simulink model "AC_Quadcopter_Simulation_2021"  (R2021b)
settings: Solver=FixedStepAuto  StartTime=0  StopTime=50  FixedStep=0.01  MaxStep=0.06  RelTol=1e-3  EnableMultiTasking=on
InitFcn:
  | kp_roll = 2.15;
  | kd_roll = 2.5;
  | 
  | Kpmin_roll = 0.9*kp_roll;
  | Kpmax_roll = 1.05*kp_roll;
  | Kdmin_roll = 0.9*kd_roll;
  | Kdmax_roll = 1.05*kd_roll;
  | 
  | kp_pitch = 2.9;
  | kd_pitch = 3.1;
  | 
  | Kpmin_pitch = 0.9*kp_pitch;
  | Kpmax_pitch = 1.05*kp_pitch;
  | Kdmin_pitch = 0.9*kd_pitch;
  | Kdmax_pitch = 1.05*kd_pitch;
  | 
  | kp_yaw = 1;
  | kd_yaw = 2.5;
  | 
  | Kpmin_yaw = 0.8*kp_yaw;
  | Kpmax_yaw = 1.2*kp_yaw;
  | Kdmin_yaw = 0.90*kd_yaw;
  | Kdmax_yaw = 1.2*kd_yaw;
StopFcn:
  | % --- FINAL Plotting Script with Angles in Degrees ---
  | 
  | disp('Generating state tracking plots with angles in degrees...');
  | 
  | try
  |     % Assuming your timeseries variable is named 'simout'
  |     timeVector = simout.Time;
  |     dataMatrix = simout.Data;
  | 
  |     % Radian to degree conversion factor
  |     rad_to_deg = 180 / pi;
  | 
  |     % Create a new, maximized figure window for the plots
  |     figure('Name', 'Quadcopter State Tracking Performance (Degrees)', 'WindowState', 'maximized');
  | 
  |     % --- 1. Roll Tracking Plot ---
  |     subplot(2, 2, 1);
  |     hold on;
  |     % Plotting Desired (Column 5) vs. Actual (Column 1)
  |     plot(timeVector, dataMatrix(:, 5) * rad_to_deg, '--', 'LineWidth', 2);
  |     plot(timeVector, dataMatrix(:, 1) * rad_to_deg, '-', 'LineWidth', 1.5);
  |     hold off;
  |     grid on;
  |     title('Roll Angle Tracking (\phi)');
  |     xlabel('Time (s)');
  |     ylabel('Angle (deg)');
  |     legend('Desired Roll (\phi_d)', 'Actual Roll (\phi)', 'Location', 'southeast');
  | 
  |     % --- 2. Pitch Tracking Plot ---
  |     subplot(2, 2, 2);
  |     hold on;
  |     % Plotting Desired (Column 6) vs. Actual (Column 2)
  |     plot(timeVector, dataMatrix(:, 6) * rad_to_deg, '--', 'LineWidth', 2);
  |     plot(timeVector, dataMatrix(:, 2) * rad_to_deg, '-', 'LineWidth', 1.5);
  |     hold off;
  |     grid on;
  |     title('Pitch Angle Tracking (\theta)');
  |     xlabel('Time (s)');
  |     ylabel('Angle (deg)');
  |     legend('Desired Pitch (\theta_d)', 'Actual Pitch (\theta)', 'Location', 'southeast');
  | 
  |     % --- 3. Yaw Tracking Plot ---
  |     subplot(2, 2, 3);
  |     hold on;
  |     % Plotting Desired (Column 7) vs. Actual (Column 3)
  |     plot(timeVector, dataMatrix(:, 7) * rad_to_deg, '--', 'LineWidth', 2);
  |     plot(timeVector, dataMatrix(:, 3) * rad_to_deg, '-', 'LineWidth', 1.5);
  |     hold off;
  |     grid on;
  |     title('Yaw Angle Tracking (\psi)');
  |     xlabel('Time (s)');
  |     ylabel('Angle (deg)');
  |     legend('Desired Yaw (\psi_d)', 'Actual Yaw (\psi)', 'Location', 'southeast');
  | 
  |     % --- 4. Altitude Tracking Plot ---
  |     subplot(2, 2, 4);
  |     hold on;
  |     % Plotting Desired (Column 8) vs. Actual (Column 4)
  |     plot(timeVector, dataMatrix(:, 8), '--', 'LineWidth', 2);
  |     plot(timeVector, dataMatrix(:, 4), '-', 'LineWidth', 1.5);
  |     hold off;
  |     grid on;
  |     title('Altitude Tracking (Z)');
  |     xlabel('Time (s)');
  |     ylabel('Position (m)');
  |     legend('Desired Altitude (Z_d)', 'Actual Altitude (Z)', 'Location', 'southeast');
  | 
  |     sgtitle('Quadcopter State Tracking Performance', 'FontSize', 16, 'FontWeight', 'bold');
  |     disp('Plots generated successfully with units in degrees.');
  | 
  | catch ME
  |     warning('Error during plotting: %s', ME.message);
  |     warning('Please ensure the variable ''simout'' exists in the workspace.');
  | end
model workspace (MAT data in the model file):
  Sig = Simulink.Signal
  Sig.DataType = 'auto'
  Sig.Dimensions = -1
  Sig.DimensionsMode = 'auto'
  Sig.Complexity = 'auto'
  Sig.SampleTime = -1
  Sig.SamplingMode = 'auto'
undefined symbols (not defined in the file): IC, quadModel
libraries: simulink x4, fuzblock x3, slpidlib x3
Description:
  | This is a configurable quadcopter simulation.
  | This Simulink model demonstates attitude control.
  | 
  | Additional quadcopter modeling and simulation materials available at:
  | github.com/dch33/Quad-Sim
  | 
  | Copyright (C) 2014 D. Hartman, K. Landis, S. Moreno, J. Kim, M. Mehrer
  | 
  | License:
  |     This program is free software: you can redistribute it and/or modify
  |     it under the terms of the GNU LESSER GENERAL PUBLIC LICENSE as published by
  |     the Free Software Foundation, either version 3 of the License, or
  |     (at your option) any later version.
  | 
  |     This program is distributed in the hope that it will be useful,
  |     but WITHOUT ANY WARRANTY; without even the implied warranty of
  |     MERCHANTABILITY or FITNESS FOR A PARTICULAR PURPOSE.  See the
  |     GNU General Public License for more details.
  | 
  |     You should have received a copy of the GNU LESSER GENERAL PUBLIC LICENSE
  |     along with this program.  If not, see <http://www.gnu.org/licenses/>.
settings Model: ModifiedComment=hp -- Sun Aug 31 10:33:41 2025 -- Version 21.0  Creator=David Hartman  LastModifiedBy=hp
settings Model: ModifiedHistory=|
  | hp -- Sun Aug 31 10:33:41 2025 -- Version 21.0
  | 
  | davidhartman -- Fri Jun 06 23:19:51 2014 -- Version 1.5
  | 
  | 
  | davidhartman -- Fri Jun 06 22:53:10 2014 -- Version 1.3
settings SolverCC: AlgebraicLoopSolver=TrustRegion  AutoInsertRateTranBlk=on
settings DataIOCC: SaveFormat=Array  SignalLogging=off  ReturnWorkspaceOutputs=off
settings OptimizationCC: DefaultParameterBehavior=Inlined  LifeSpan=inf
settings DebuggingCC: UnderspecifiedInitializationDetection=Classic  MergeDetectMultiDrivingBlocksExec=none  SolverPrmCheckMsg=warning  UniqueDataStoreMsg=warning  StateNameClashWarn=warning  StrictBusMsg=WarnOnBusTreatedAsVector  SFUnexpectedBacktrackingDiag=warning  SFNoUnconditionalDefaultTransitionDiag=warning  SFExecutionAtInitializationDiag=none  ArithmeticOperatorsInVariantConditions=warning
settings HardwareCC: ProdBitPerPointer=32  ProdBitPerSizeT=32  ProdBitPerPtrDiffT=32  ProdLargestAtomicFloat=None  ProdIntDivRoundTo=Undefined  ProdEndianess=Unspecified  ProdWordSize=32  ProdHWDeviceType=32-bit Generic
settings ModelReferenceCC: EnableRefExpFcnMdlSchedulingChecks=off  PropagateSignalLabelsOutOfModel=off
settings SFSimCC: SimUseLocalCustomCode=off  CustomCodeUndefinedFunction=UseInterfaceOnly
settings RTWCC: RTWUseLocalCustomCode=off  DLArmComputeVersion=20.02.1
settings CodeAppCC: StateflowObjectComments=on
settings GRTTargetCC: TargetLangStandard=C89/C90 (ANSI)
settings ConfigComp: CovMetricSettings=dw  CovSaveCumulativeToWorkspaceVar=on  CovSaveSingleToWorkspaceVar=on  CovExternalEMLEnable=off

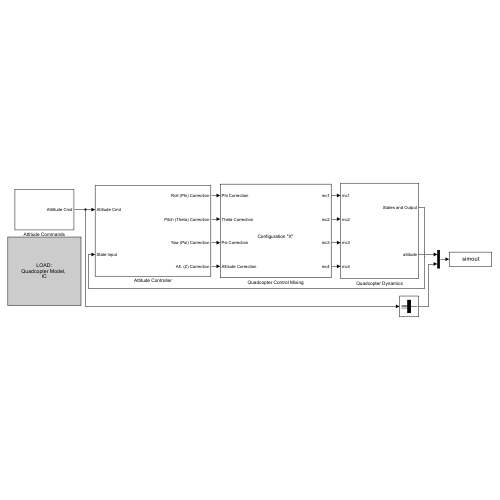
[thumbnail: Simulink's stored preview of the top-level diagram]
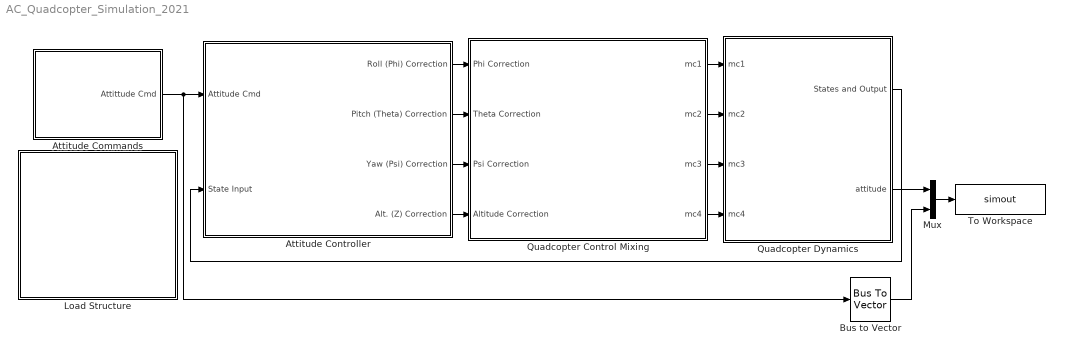
== system AC_Quadcopter_Simulation_2021 ==
  Attitude Commands : Subsystem
  Attitude Controller : Subsystem
  Bus to Vector : BusToVector
  Load Structure : Subsystem
      settings: OpenFcn=|
      | uiopen('load')
      | if ((exist('IC')==1) && (exist('quadModel')==1) && (exist('path')==1))
      | set_param(bdroot, 'SimulationCommand', 'update')
      | end
      mask Display: fprintf('LOAD:\nQuadcopter Model, \nIC')
  Mux : Mux  Inputs=2
  Quadcopter Control Mixing : Subsystem
      mask Display:
      | modelLoaded = evalin('base','exist(''quadModel'',''var'')');
      | if (modelLoaded==1)
      |     if (evalin('base','quadModel.plusConfig'))
      |     fprintf([' \n' ' \n'  'Configuration "+"']);
      |     else if (~evalin('base','quadModel.plusConfig'))
      |         fprintf([' \n' ' \n' 'Configuration "X"']);
      |         end
      |     end
      | else
      |     fprintf([' \n' ' \n'  'Model Not Loaded']);
      | end
  Quadcopter Dynamics : Subsystem
  To Workspace : ToWorkspace  VariableName=simout  SaveFormat=Timeseries  SampleTime=-1
  wires:
  Quadcopter Control Mixing/1(mc1) -> Quadcopter Dynamics/1(mc1)
  Quadcopter Dynamics/1(States and Output) -> Attitude Controller/2(State Input)
  Quadcopter Control Mixing/4(mc4) -> Quadcopter Dynamics/4(mc4)
  Quadcopter Control Mixing/2(mc2) -> Quadcopter Dynamics/2(mc2)
  Quadcopter Control Mixing/3(mc3) -> Quadcopter Dynamics/3(mc3)
  Attitude Commands/1(Attittude Cmd) -> Bus to Vector/1, Attitude Controller/1(Attitude Cmd)
  Attitude Controller/1(Roll (Phi) Correction) -> Quadcopter Control Mixing/1(Phi Correction)
  Attitude Controller/2(Pitch (Theta) Correction) -> Quadcopter Control Mixing/2(Theta Correction)
  Attitude Controller/3(Yaw (Psi) Correction) -> Quadcopter Control Mixing/3(Psi Correction)
  Attitude Controller/4(Alt. (Z) Correction) -> Quadcopter Control Mixing/4(Altitude Correction)
  Quadcopter Dynamics/2(attitude) -> Mux/1
  Mux/1 -> To Workspace/1
  Bus to Vector/1 -> Mux/2

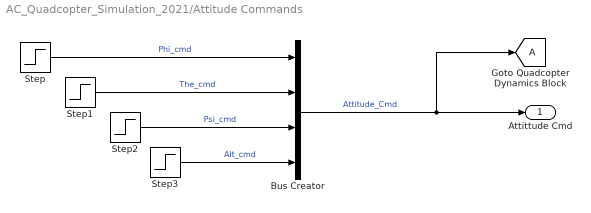
== system AC_Quadcopter_Simulation_2021/Attitude Commands ==
  Bus Creator : BusCreator  Inputs=4
  Step : Step  Time=4  After=-10*pi/180  SampleTime=0
  Step1 : Step  After=10*pi/180  SampleTime=0
  Step2 : Step  Time=7  After=45*pi/180  SampleTime=0
  Step3 : Step  Time=0  Before=10*0.3048  After=10*0.3048  SampleTime=0
  Attittude Cmd : Outport
  tag scope: A=global
  wires:
  Bus Creator/1 -> Attittude Cmd/1, [A]  "Attitude_Cmd"
  Step3/1 -> Bus Creator/4  "Alt_cmd"
  Step2/1 -> Bus Creator/3  "Psi_cmd"
  Step1/1 -> Bus Creator/2  "The_cmd"
  Step/1 -> Bus Creator/1  "Phi_cmd"

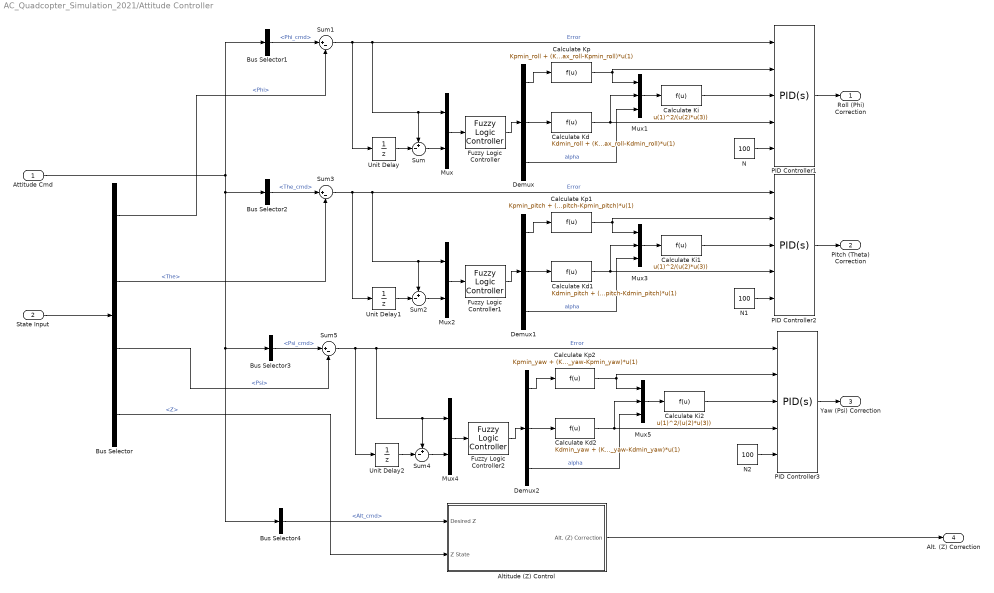
== system AC_Quadcopter_Simulation_2021/Attitude Controller ==
  Attitude Cmd : Inport
  State Input : Inport  Port=2
  Altitude (Z) Control : Subsystem  mask{Kpz=2, Kiz=1.1, Kdz=3.3, LimitOutput=on, USat=1, LSat=-1, GOffset=(sqrt((quadModel.mass*quadModel.g)/(4*quadModel.ct))-quadModel.b)/quadModel.cr}
      mask prompts: Kpz "Kp"; Kiz "Ki"; Kdz "Kd"; LimitOutput "Integral Saturation?"; USat "Upper saturation limit:"; LSat "Lower saturation limit:"; GOffset "Gravity Feedforward"
      mask help:
      | Adjust PID controller gains through this mask interface, or "look under mask" for more detailed adjustments.
      |
      | Note: Gravity Offset will not appear on block face as a value until simulation is run if it is the result of a formula involving the quadcopter model parameters.
      mask TypeOptions Kpz: Kpz/Gain
      mask TypeOptions Kiz: Kiz/Gain
      mask TypeOptions Kdz: Kdz/Gain
      mask TypeOptions LimitOutput:
      | Integrator
      | Limited/LimitOutput
      mask TypeOptions USat:
      | Integrator
      | Limited/UpperSaturationLimit
      mask TypeOptions LSat:
      | Integrator
      | Limited/LowerSaturationLimit
      mask TypeOptions GOffset: Gravity Offset (Level Flight)/Value
      mask Display:
      | fprintf(['Kp = ' num2str(Kpz) '\n' ...
      |     'Ki = ' num2str(Kiz) '\n' ...
      |     'Kd = ' num2str(Kdz) '\n' ...
      |     'Integral Saturation: ' LimitOutput]);
      | if strcmp(LimitOutput,'on')
      |     fprintf([' \n' ' \n' ' \n' ' \n' ' \n' '\n' ...
      |         'Limits: ' num2str(USat) ' to ' num2str(LSat)]);
      | end
  Bus Selector : BusSelector  OutputSignals=Phi,The,Psi,Z
  Bus Selector1 : BusSelector  OutputSignals=Phi_cmd
  Bus Selector2 : BusSelector  OutputSignals=The_cmd
  Bus Selector3 : BusSelector  OutputSignals=Psi_cmd
  Bus Selector4 : BusSelector  OutputSignals=Alt_cmd
  Calculate Kd : Fcn  Expr=Kdmin_roll + (Kdmax_roll-Kdmin_roll)*u(1)
  Calculate Kd1 : Fcn  Expr=Kdmin_pitch + (Kdmax_pitch-Kdmin_pitch)*u(1)
  Calculate Kd2 : Fcn  Expr=Kdmin_yaw + (Kdmax_yaw-Kdmin_yaw)*u(1)
  Calculate Ki : Fcn  Expr=u(1)^2/(u(2)*u(3))
  Calculate Ki1 : Fcn  Expr=u(1)^2/(u(2)*u(3))
  Calculate Ki2 : Fcn  Expr=u(1)^2/(u(2)*u(3))
  Calculate Kp : Fcn  Expr=Kpmin_roll + (Kpmax_roll-Kpmin_roll)*u(1)
  Calculate Kp1 : Fcn  Expr=Kpmin_pitch + (Kpmax_pitch-Kpmin_pitch)*u(1)
  Calculate Kp2 : Fcn  Expr=Kpmin_yaw + (Kpmax_yaw-Kpmin_yaw)*u(1)
  Demux : Demux  Outputs=3
  Demux1 : Demux  Outputs=3
  Demux2 : Demux  Outputs=3
  Fuzzy Logic Controller : fuzblock/Fuzzy Logic  Controller  FIS='PID_Fuzzy.fis'  OutputSampleNumber=101  DataType=double  FuzzifiedInputs=off  RuleFiringStrengths=off  RuleOutputs=off  AggregatedOutputs=off  SimulateUsing=Interpreted execution  OutOfRangeInputValueMessage=warning  NoRuleFiredMessage=warning  EmptyOutputFuzzySetMessage=warning
  Fuzzy Logic Controller1 : fuzblock/Fuzzy Logic  Controller  FIS='PID_Fuzzy.fis'  OutputSampleNumber=101  DataType=double  FuzzifiedInputs=off  RuleFiringStrengths=off  RuleOutputs=off  AggregatedOutputs=off  SimulateUsing=Interpreted execution  OutOfRangeInputValueMessage=warning  NoRuleFiredMessage=warning  EmptyOutputFuzzySetMessage=warning
  Fuzzy Logic Controller2 : fuzblock/Fuzzy Logic  Controller  FIS='PID_Fuzzy.fis'  OutputSampleNumber=101  DataType=double  FuzzifiedInputs=off  RuleFiringStrengths=off  RuleOutputs=off  AggregatedOutputs=off  SimulateUsing=Interpreted execution  OutOfRangeInputValueMessage=warning  NoRuleFiredMessage=warning  EmptyOutputFuzzySetMessage=warning
  Mux : Mux  Inputs=2
  Mux1 : Mux  Inputs=3
  Mux2 : Mux  Inputs=2
  Mux3 : Mux  Inputs=3
  Mux4 : Mux  Inputs=2
  Mux5 : Mux  Inputs=3
  N : Constant  Value=100
  N1 : Constant  Value=100
  N2 : Constant  Value=100
  PID Controller1 : slpidlib/PID Controller  Controller=PID  Form=Parallel  TimeDomain=Continuous-time  UseExternalTs=off  SampleTime=-1  IntegratorMethod=Forward Euler  FilterMethod=Forward Euler  ControllerParametersSource=external  P=0.6*4.6737  I=1.2*4.6737/3.26  D=0.6*4.6737*3.26/8  N=100  UseFilter=on  TunerSelectOption=Transfer Function Based (PID Tuner App)  InitialConditionSource=internal  InitialConditionForIntegrator=0  InitialConditionForFilter=0  DifferentiatorICPrevScaledInput=0  ExternalReset=none  TrackingMode=off  Kt=1  LimitOutput=off  SatLimitsSource=internal  UpperSaturationLimit=inf  LowerSaturationLimit=-inf  LinearizeAsGain=on  AntiWindupMode=none  Kb=1  POutMin=[]  POutMax=[]  IOutMin=[]  IOutMax=[]  DOutMin=[]  DOutMax=[]  NOutMin=[]  NOutMax=[]  SumOutMin=[]  SumOutMax=[]  SaturationOutMin=[]  SaturationOutMax=[]  PParamMin=[]  PParamMax=[]  IParamMin=[]  IParamMax=[]  DParamMin=[]  DParamMax=[]  NParamMin=[]  NParamMax=[]  KbParamMin=[]  KbParamMax=[]  KtParamMin=[]  KtParamMax=[]  KbOutMin=[]  KbOutMax=[]  KtOutMin=[]  KtOutMax=[]  IntegratorOutMin=[]  IntegratorOutMax=[]  FilterOutMin=[]  FilterOutMax=[]  SumI1OutMin=[]  SumI1OutMax=[]  SumI2OutMin=[]  SumI2OutMax=[]  SumI3OutMin=[]  SumI3OutMax=[]  SumI4OutMin=[]  SumI4OutMax=[]  SumDOutMin=[]  SumDOutMax=[]  DifferentiatorOutMin=[]  DifferentiatorOutMax=[]  FilterDiffOutCoefMin=[]  FilterDiffOutCoefMax=[]  ReciprocalOutMin=[]  ReciprocalOutMax=[]  SumDenOutMin=[]  SumDenOutMax=[]  SumNumOutMin=[]  SumNumOutMax=[]  DivideOutMin=[]  DivideOutMax=[]  UdiffTsProdOutMin=[]  UdiffTsProdOutMax=[]  NTsProdOutMin=[]  NTsProdOutMax=[]  UintegralTsProdOutMin=[]  UintegralTsProdOutMax=[]  UngainTsProdOutMin=[]  UngainTsProdOutMax=[]  IntegratorContinuousStateAttributes=''  IntegratorStateMustResolveToSignalObject=off  IntegratorRTWStateStorageClass=Auto  FilterContinuousStateAttributes=''  FilterStateMustResolveToSignalObject=off  FilterRTWStateStorageClass=Auto  ParallelPVariant=ExternalParameters  IdealPVariant=Disabled  IVariant=ExternalParameters  DVariant=ExternalParameters  IntegratorVariant=Continuous  SatVariant=Disabled  AWVariant=Passthrough  PCopyVariant=Disabled  TRVariant=Disabled  FdbkBlocksVariant=Forward  IdealPFdbkVariant=Disabled  SatFdbkVariant=Disabled  DerivativeFilterVariant=ContFilter  NVariant=ExternalParameters  NCopyVariant=Disabled  FilterICVariant=InternalICsFilter  IntegratorICVariant=InternalICs  ExternalResetVariant=Disabled  TRSumVariant=Passthrough  SumFdbkVariant=Disabled  SumVariant=Sum_PID  TsampFilterVariant=InternalTs  TsampNgainVariant=Passthrough  TsampIntegralVariant=Disabled_SignalSpec  ExternalSaturationOutDataTypeStr=Inherit: Same as second input
  PID Controller2 : slpidlib/PID Controller  Controller=PID  Form=Parallel  TimeDomain=Continuous-time  UseExternalTs=off  SampleTime=-1  IntegratorMethod=Forward Euler  FilterMethod=Forward Euler  ControllerParametersSource=external  P=0.6*4.6737  I=1.2*4.6737/3.26  D=0.6*4.6737*3.26/8  N=100  UseFilter=on  TunerSelectOption=Transfer Function Based (PID Tuner App)  InitialConditionSource=internal  InitialConditionForIntegrator=0  InitialConditionForFilter=0  DifferentiatorICPrevScaledInput=0  ExternalReset=none  TrackingMode=off  Kt=1  LimitOutput=off  SatLimitsSource=internal  UpperSaturationLimit=inf  LowerSaturationLimit=-inf  LinearizeAsGain=on  AntiWindupMode=none  Kb=1  POutMin=[]  POutMax=[]  IOutMin=[]  IOutMax=[]  DOutMin=[]  DOutMax=[]  NOutMin=[]  NOutMax=[]  SumOutMin=[]  SumOutMax=[]  SaturationOutMin=[]  SaturationOutMax=[]  PParamMin=[]  PParamMax=[]  IParamMin=[]  IParamMax=[]  DParamMin=[]  DParamMax=[]  NParamMin=[]  NParamMax=[]  KbParamMin=[]  KbParamMax=[]  KtParamMin=[]  KtParamMax=[]  KbOutMin=[]  KbOutMax=[]  KtOutMin=[]  KtOutMax=[]  IntegratorOutMin=[]  IntegratorOutMax=[]  FilterOutMin=[]  FilterOutMax=[]  SumI1OutMin=[]  SumI1OutMax=[]  SumI2OutMin=[]  SumI2OutMax=[]  SumI3OutMin=[]  SumI3OutMax=[]  SumI4OutMin=[]  SumI4OutMax=[]  SumDOutMin=[]  SumDOutMax=[]  DifferentiatorOutMin=[]  DifferentiatorOutMax=[]  FilterDiffOutCoefMin=[]  FilterDiffOutCoefMax=[]  ReciprocalOutMin=[]  ReciprocalOutMax=[]  SumDenOutMin=[]  SumDenOutMax=[]  SumNumOutMin=[]  SumNumOutMax=[]  DivideOutMin=[]  DivideOutMax=[]  UdiffTsProdOutMin=[]  UdiffTsProdOutMax=[]  NTsProdOutMin=[]  NTsProdOutMax=[]  UintegralTsProdOutMin=[]  UintegralTsProdOutMax=[]  UngainTsProdOutMin=[]  UngainTsProdOutMax=[]  IntegratorContinuousStateAttributes=''  IntegratorStateMustResolveToSignalObject=off  IntegratorRTWStateStorageClass=Auto  FilterContinuousStateAttributes=''  FilterStateMustResolveToSignalObject=off  FilterRTWStateStorageClass=Auto  ParallelPVariant=ExternalParameters  IdealPVariant=Disabled  IVariant=ExternalParameters  DVariant=ExternalParameters  IntegratorVariant=Continuous  SatVariant=Disabled  AWVariant=Passthrough  PCopyVariant=Disabled  TRVariant=Disabled  FdbkBlocksVariant=Forward  IdealPFdbkVariant=Disabled  SatFdbkVariant=Disabled  DerivativeFilterVariant=ContFilter  NVariant=ExternalParameters  NCopyVariant=Disabled  FilterICVariant=InternalICsFilter  IntegratorICVariant=InternalICs  ExternalResetVariant=Disabled  TRSumVariant=Passthrough  SumFdbkVariant=Disabled  SumVariant=Sum_PID  TsampFilterVariant=InternalTs  TsampNgainVariant=Passthrough  TsampIntegralVariant=Disabled_SignalSpec  ExternalSaturationOutDataTypeStr=Inherit: Same as second input
  PID Controller3 : slpidlib/PID Controller  Controller=PID  Form=Parallel  TimeDomain=Continuous-time  UseExternalTs=off  SampleTime=-1  IntegratorMethod=Forward Euler  FilterMethod=Forward Euler  ControllerParametersSource=external  P=0.6*4.6737  I=1.2*4.6737/3.26  D=0.6*4.6737*3.26/8  N=100  UseFilter=on  TunerSelectOption=Transfer Function Based (PID Tuner App)  InitialConditionSource=internal  InitialConditionForIntegrator=0  InitialConditionForFilter=0  DifferentiatorICPrevScaledInput=0  ExternalReset=none  TrackingMode=off  Kt=1  LimitOutput=off  SatLimitsSource=internal  UpperSaturationLimit=inf  LowerSaturationLimit=-inf  LinearizeAsGain=on  AntiWindupMode=none  Kb=1  POutMin=[]  POutMax=[]  IOutMin=[]  IOutMax=[]  DOutMin=[]  DOutMax=[]  NOutMin=[]  NOutMax=[]  SumOutMin=[]  SumOutMax=[]  SaturationOutMin=[]  SaturationOutMax=[]  PParamMin=[]  PParamMax=[]  IParamMin=[]  IParamMax=[]  DParamMin=[]  DParamMax=[]  NParamMin=[]  NParamMax=[]  KbParamMin=[]  KbParamMax=[]  KtParamMin=[]  KtParamMax=[]  KbOutMin=[]  KbOutMax=[]  KtOutMin=[]  KtOutMax=[]  IntegratorOutMin=[]  IntegratorOutMax=[]  FilterOutMin=[]  FilterOutMax=[]  SumI1OutMin=[]  SumI1OutMax=[]  SumI2OutMin=[]  SumI2OutMax=[]  SumI3OutMin=[]  SumI3OutMax=[]  SumI4OutMin=[]  SumI4OutMax=[]  SumDOutMin=[]  SumDOutMax=[]  DifferentiatorOutMin=[]  DifferentiatorOutMax=[]  FilterDiffOutCoefMin=[]  FilterDiffOutCoefMax=[]  ReciprocalOutMin=[]  ReciprocalOutMax=[]  SumDenOutMin=[]  SumDenOutMax=[]  SumNumOutMin=[]  SumNumOutMax=[]  DivideOutMin=[]  DivideOutMax=[]  UdiffTsProdOutMin=[]  UdiffTsProdOutMax=[]  NTsProdOutMin=[]  NTsProdOutMax=[]  UintegralTsProdOutMin=[]  UintegralTsProdOutMax=[]  UngainTsProdOutMin=[]  UngainTsProdOutMax=[]  IntegratorContinuousStateAttributes=''  IntegratorStateMustResolveToSignalObject=off  IntegratorRTWStateStorageClass=Auto  FilterContinuousStateAttributes=''  FilterStateMustResolveToSignalObject=off  FilterRTWStateStorageClass=Auto  ParallelPVariant=ExternalParameters  IdealPVariant=Disabled  IVariant=ExternalParameters  DVariant=ExternalParameters  IntegratorVariant=Continuous  SatVariant=Disabled  AWVariant=Passthrough  PCopyVariant=Disabled  TRVariant=Disabled  FdbkBlocksVariant=Forward  IdealPFdbkVariant=Disabled  SatFdbkVariant=Disabled  DerivativeFilterVariant=ContFilter  NVariant=ExternalParameters  NCopyVariant=Disabled  FilterICVariant=InternalICsFilter  IntegratorICVariant=InternalICs  ExternalResetVariant=Disabled  TRSumVariant=Passthrough  SumFdbkVariant=Disabled  SumVariant=Sum_PID  TsampFilterVariant=InternalTs  TsampNgainVariant=Passthrough  TsampIntegralVariant=Disabled_SignalSpec  ExternalSaturationOutDataTypeStr=Inherit: Same as second input
  Sum : Sum  Inputs=+-|
  Sum1 : Sum  Inputs=|+-
  Sum2 : Sum  Inputs=+-|
  Sum3 : Sum  Inputs=|+-
  Sum4 : Sum  Inputs=+-|
  Sum5 : Sum  Inputs=|+-
  Unit Delay : UnitDelay  SampleTime=-1  HasFrameUpgradeWarning=on
  Unit Delay1 : UnitDelay  SampleTime=-1  HasFrameUpgradeWarning=on
  Unit Delay2 : UnitDelay  SampleTime=-1  HasFrameUpgradeWarning=on
  Roll (Phi) Correction : Outport
  Pitch (Theta) Correction : Outport  Port=2
  Yaw (Psi) Correction : Outport  Port=3
  Alt. (Z) Correction : Outport  Port=4
  wires:
  State Input/1 -> Bus Selector/1
  Bus Selector/1 -> Sum1/2  "<Phi>"
  Calculate Ki/1 -> PID Controller1/3
  Fuzzy Logic Controller/1 -> Demux/1
  Demux/2 -> Calculate Kd/1
  Mux1/1 -> Calculate Ki/1
  N/1 -> PID Controller1/5
  PID Controller1/1 -> Roll (Phi) Correction/1
  Mux/1 -> Fuzzy Logic Controller/1
  Demux/1 -> Calculate Kp/1
  Calculate Kp/1 -> PID Controller1/2, Mux1/1
  Unit Delay/1 -> Sum/2
  Sum/1 -> Mux/2
  Demux/3 -> Mux1/3  "alpha"
  Sum1/1 -> Unit Delay/1, PID Controller1/1, Sum/1, Mux/1  "Error"
  Bus Selector1/1 -> Sum1/1  "<Phi_cmd>"
  Calculate Kd1/1 -> Mux3/2, PID Controller2/4
  Demux1/3 -> Mux3/3  "alpha"
  Unit Delay1/1 -> Sum2/2
  Sum2/1 -> Mux2/2
  Calculate Kp1/1 -> PID Controller2/2, Mux3/1
  Calculate Ki1/1 -> PID Controller2/3
  N1/1 -> PID Controller2/5
  Demux1/1 -> Calculate Kp1/1
  Demux1/2 -> Calculate Kd1/1
  Sum3/1 -> Unit Delay1/1, PID Controller2/1, Sum2/1, Mux2/1  "Error"
  Mux2/1 -> Fuzzy Logic Controller1/1
  Bus Selector2/1 -> Sum3/1  "<The_cmd>"
  Mux3/1 -> Calculate Ki1/1
  Fuzzy Logic Controller1/1 -> Demux1/1
  Bus Selector/2 -> Sum3/2  "<The>"
  PID Controller2/1 -> Pitch (Theta) Correction/1
  Sum5/1 -> Unit Delay2/1, PID Controller3/1, Sum4/1, Mux4/1  "Error"
  Calculate Ki2/1 -> PID Controller3/3
  N2/1 -> PID Controller3/5
  Unit Delay2/1 -> Sum4/2
  Sum4/1 -> Mux4/2
  Demux2/1 -> Calculate Kp2/1
  Demux2/2 -> Calculate Kd2/1
  Demux2/3 -> Mux5/3  "alpha"
  Bus Selector3/1 -> Sum5/1  "<Psi_cmd>"
  Calculate Kd2/1 -> Mux5/2, PID Controller3/4
  Fuzzy Logic Controller2/1 -> Demux2/1
  Mux4/1 -> Fuzzy Logic Controller2/1
  Calculate Kp2/1 -> PID Controller3/2, Mux5/1
  Mux5/1 -> Calculate Ki2/1
  Bus Selector/3 -> Sum5/2  "<Psi>"
  PID Controller3/1 -> Yaw (Psi) Correction/1
  Attitude Cmd/1 -> Bus Selector4/1, Bus Selector3/1, Bus Selector2/1, Bus Selector1/1
  Altitude (Z) Control/1(Alt. (Z) Correction) -> Alt. (Z) Correction/1
  Bus Selector4/1 -> Altitude (Z) Control/1(Desired Z)  "<Alt_cmd>"
  Bus Selector/4 -> Altitude (Z) Control/2(Z State)  "<Z>"
  Calculate Kd/1 -> Mux1/2, PID Controller1/4

== system AC_Quadcopter_Simulation_2021/Load Structure ==

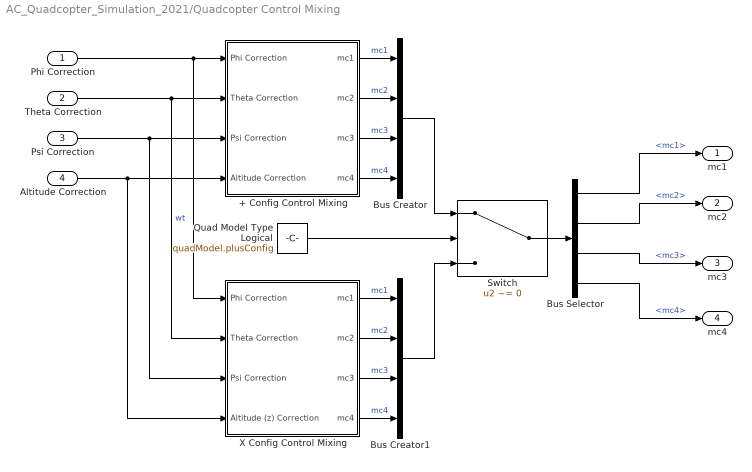
== system AC_Quadcopter_Simulation_2021/Quadcopter Control Mixing ==
  Phi Correction : Inport
  Theta Correction : Inport  Port=2
  Psi Correction : Inport  Port=3
  Altitude Correction : Inport  Port=4
  + Config Control Mixing : Subsystem
  Bus Creator : BusCreator  Inputs=4
  Bus Creator1 : BusCreator  Inputs=4
  Bus Selector : BusSelector  OutputSignals=mc1,mc2,mc3,mc4
  Quad Model Type Logical : Constant  Value=quadModel.plusConfig
  Switch : Switch  Criteria=u2 ~= 0
  X Config Control Mixing : Subsystem
  mc1 : Outport
  mc2 : Outport  Port=2
  mc3 : Outport  Port=3
  mc4 : Outport  Port=4
  wires:
  Switch/1 -> Bus Selector/1
  Quad Model Type Logical/1 -> Switch/2
  Bus Selector/4 -> mc4/1  "<mc4>"
  Bus Selector/3 -> mc3/1  "<mc3>"
  Bus Selector/2 -> mc2/1  "<mc2>"
  Bus Selector/1 -> mc1/1  "<mc1>"
  Bus Creator1/1 -> Switch/3
  X Config Control Mixing/4(mc4) -> Bus Creator1/4  "mc4"
  X Config Control Mixing/3(mc3) -> Bus Creator1/3  "mc3"
  X Config Control Mixing/2(mc2) -> Bus Creator1/2  "mc2"
  X Config Control Mixing/1(mc1) -> Bus Creator1/1  "mc1"
  Bus Creator/1 -> Switch/1
  + Config Control Mixing/4(mc4) -> Bus Creator/4  "mc4"
  + Config Control Mixing/3(mc3) -> Bus Creator/3  "mc3"
  + Config Control Mixing/2(mc2) -> Bus Creator/2  "mc2"
  + Config Control Mixing/1(mc1) -> Bus Creator/1  "mc1"
  Altitude Correction/1 -> + Config Control Mixing/4(Altitude Correction), X Config Control Mixing/4(Altitude (z) Correction)
  Psi Correction/1 -> + Config Control Mixing/3(Psi Correction), X Config Control Mixing/3(Psi Correction)
  Theta Correction/1 -> + Config Control Mixing/2(Theta Correction), X Config Control Mixing/2(Theta Correction)  "wt"
  Phi Correction/1 -> + Config Control Mixing/1(Phi Correction), X Config Control Mixing/1(Phi Correction)

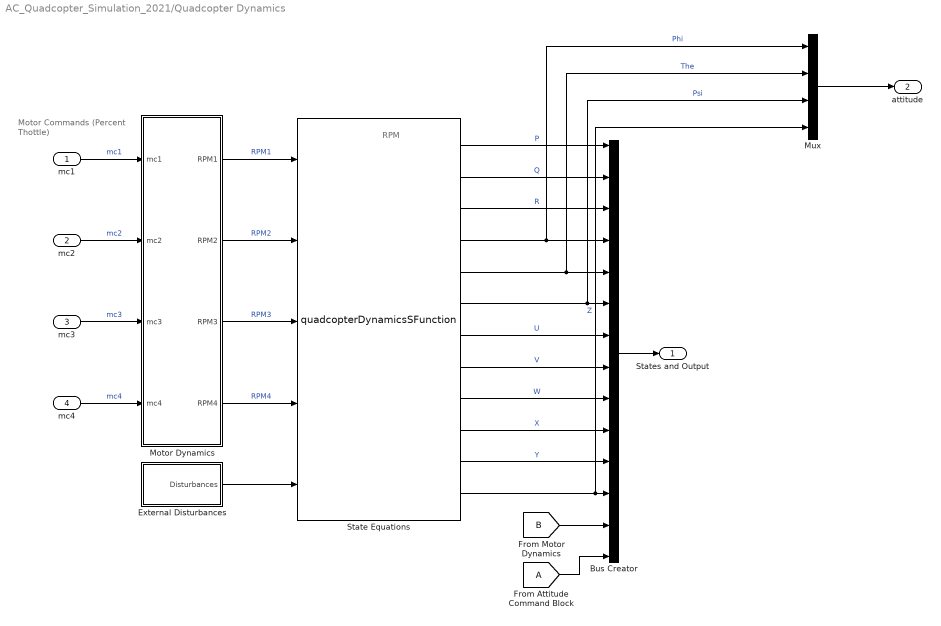
== system AC_Quadcopter_Simulation_2021/Quadcopter Dynamics ==
  note: Motor Commands
      | (Percent Thottle)
  note: RPM
  mc1 : Inport
  mc2 : Inport  Port=2
  mc3 : Inport  Port=3
  mc4 : Inport  Port=4
  Bus Creator : BusCreator  Inputs='P','Q','R','Phi','The','Psi','U','V','W','X','Y','Z','mc and RPM','Attitude_Cmd'
  External Disturbances : Subsystem
  Motor Dynamics : Subsystem
  Mux : Mux
  State Equations : M-S-Function  FunctionName=quadcopterDynamicsSFunction  Parameters=quadModel, IC
      mask Display:
      | port_label('input', 1, 'RPM1')
      | port_label('input', 2, 'RPM2')
      | port_label('input', 3, 'RPM3')
      | port_label('input', 4, 'RPM4')
      | port_label('input', 5, 'Disturbances')
      | port_label('output', 1, 'P')
      | port_label('output', 2, 'Q')
      | port_label('output', 3, 'R')
      | port_label('output', 4, 'Phi')
      | port_label('output', 5, 'The')
      | port_label('output', 6, 'Psi')
      | port_label('output', 7, 'U')
      | port_label('output', 8, 'V')
      | port_label('output', 9, 'W')
      | port_label('output', 10, 'X')
      | port_label('output', 11, 'Y')
      | port_label('output', 12, 'Z')
  States and Output : Outport
  attitude : Outport  Port=2
  wires:
  [B] -> Bus Creator/13
  [A] -> Bus Creator/14
  External Disturbances/1("Disturbances ") -> State Equations/5
  mc2/1 -> Motor Dynamics/2(mc2)  "mc2"
  mc3/1 -> Motor Dynamics/3(mc3)  "mc3"
  mc4/1 -> Motor Dynamics/4(mc4)  "mc4"
  mc1/1 -> Motor Dynamics/1(mc1)  "mc1"
  Motor Dynamics/4(RPM4) -> State Equations/4  "RPM4"
  Motor Dynamics/3(RPM3) -> State Equations/3  "RPM3"
  Motor Dynamics/2(RPM2) -> State Equations/2  "RPM2"
  Motor Dynamics/1(RPM1) -> State Equations/1  "RPM1"
  State Equations/12 -> Mux/4, Bus Creator/12  "Z"
  State Equations/11 -> Bus Creator/11  "Y"
  State Equations/10 -> Bus Creator/10  "X"
  State Equations/9 -> Bus Creator/9  "W"
  State Equations/8 -> Bus Creator/8  "V"
  State Equations/7 -> Bus Creator/7  "U"
  State Equations/6 -> Mux/3, Bus Creator/6  "Psi"
  State Equations/5 -> Mux/2, Bus Creator/5  "The"
  State Equations/4 -> Mux/1, Bus Creator/4  "Phi"
  State Equations/3 -> Bus Creator/3  "R"
  State Equations/2 -> Bus Creator/2  "Q"
  State Equations/1 -> Bus Creator/1  "P"
  Mux/1 -> attitude/1
  Bus Creator/1 -> States and Output/1

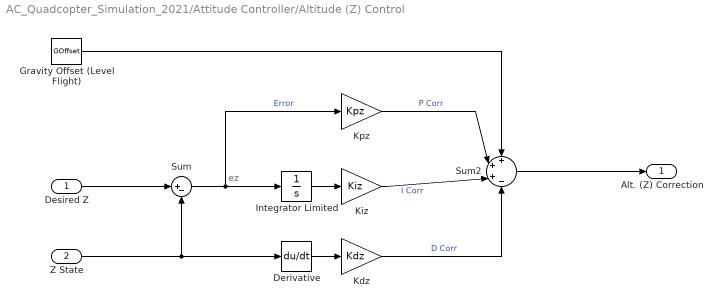
== system AC_Quadcopter_Simulation_2021/Attitude Controller/Altitude (Z) Control ==
  note: ez
  Desired Z : Inport
  Z State : Inport  Port=2
  Derivative : Derivative
  Gravity Offset (Level Flight) : Constant  Value=GOffset
  Integrator Limited : Integrator  LimitOutput=on  UpperSaturationLimit=USat  LowerSaturationLimit=LSat
  Kdz : Gain  Gain=Kdz
  Kiz : Gain  Gain=Kiz
  Kpz : Gain  Gain=Kpz
  Sum : Sum  Inputs=|+-
  Sum2 : Sum  Inputs=+++-
  Alt. (Z) Correction : Outport
  wires:
  Gravity Offset (Level Flight)/1 -> Sum2/1
  Desired Z/1 -> Sum/1
  Z State/1 -> Derivative/1, Sum/2
  Sum2/1 -> Alt. (Z) Correction/1
  Kpz/1 -> Sum2/2  "P Corr"
  Sum/1 -> Integrator Limited/1, Kpz/1  "Error"
  Kiz/1 -> Sum2/3  "I Corr"
  Kdz/1 -> Sum2/4  "D Corr"
  Integrator Limited/1 -> Kiz/1
  Derivative/1 -> Kdz/1

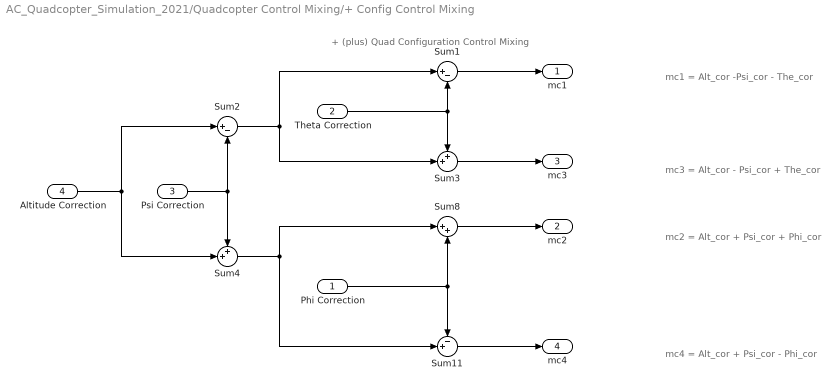
== system AC_Quadcopter_Simulation_2021/Quadcopter Control Mixing/+ Config Control Mixing ==
  note: mc1 = Alt_cor -Psi_cor - The_cor
  note: mc3 = Alt_cor - Psi_cor + The_cor
  note: mc4 = Alt_cor + Psi_cor - Phi_cor
  note: + (plus) Quad Configuration Control Mixing
  note: mc2 = Alt_cor + Psi_cor + Phi_cor
  Phi Correction : Inport
  Theta Correction : Inport  Port=2
  Psi Correction : Inport  Port=3
  Altitude Correction : Inport  Port=4
  Sum1 : Sum  Inputs=|+-
  Sum11 : Sum  Inputs=-+|
  Sum2 : Sum  Inputs=|+-
  Sum3 : Sum  Inputs=++|
  Sum4 : Sum  Inputs=++|
  Sum8 : Sum  Inputs=|++
  mc1 : Outport
  mc2 : Outport  Port=2
  mc3 : Outport  Port=3
  mc4 : Outport  Port=4
  wires:
  Sum11/1 -> mc4/1
  Sum8/1 -> mc2/1
  Sum3/1 -> mc3/1
  Sum1/1 -> mc1/1
  Phi Correction/1 -> Sum11/1, Sum8/2
  Sum4/1 -> Sum8/1, Sum11/2
  Psi Correction/1 -> Sum2/2, Sum4/1
  Sum2/1 -> Sum1/1, Sum3/2
  Altitude Correction/1 -> Sum4/2, Sum2/1
  Theta Correction/1 -> Sum3/1, Sum1/2

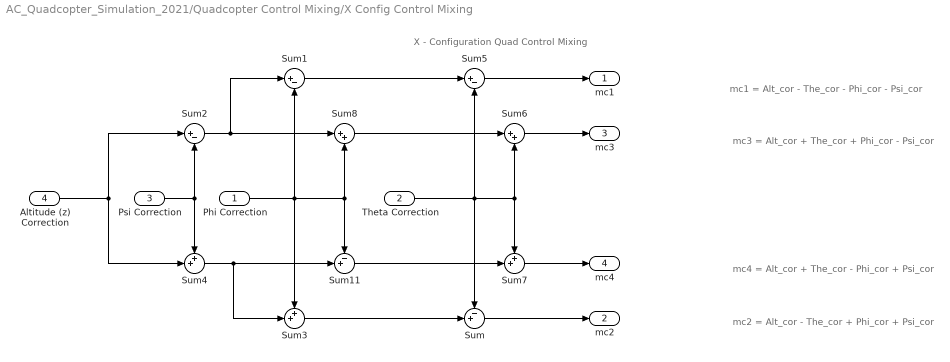
== system AC_Quadcopter_Simulation_2021/Quadcopter Control Mixing/X Config Control Mixing ==
  note: mc4 = Alt_cor + The_cor - Phi_cor + Psi_cor
  note: mc2 = Alt_cor - The_cor + Phi_cor + Psi_cor
  note: mc3 = Alt_cor + The_cor + Phi_cor - Psi_cor
  note: X - Configuration Quad Control Mixing
  note: mc1 = Alt_cor - The_cor - Phi_cor - Psi_cor
  Phi Correction : Inport
  Theta Correction : Inport  Port=2
  Psi Correction : Inport  Port=3
  Altitude (z) Correction : Inport  Port=4
  Sum : Sum  Inputs=-+|
  Sum1 : Sum  Inputs=|+-
  Sum11 : Sum  Inputs=-+|
  Sum2 : Sum  Inputs=|+-
  Sum3 : Sum  Inputs=++|
  Sum4 : Sum  Inputs=++|
  Sum5 : Sum  Inputs=|+-
  Sum6 : Sum  Inputs=|++
  Sum7 : Sum  Inputs=++|
  Sum8 : Sum  Inputs=|++
  mc1 : Outport
  mc2 : Outport  Port=2
  mc3 : Outport  Port=3
  mc4 : Outport  Port=4
  wires:
  Sum/1 -> mc2/1
  Altitude (z) Correction/1 -> Sum4/2, Sum2/1
  Sum7/1 -> mc4/1
  Sum6/1 -> mc3/1
  Sum5/1 -> mc1/1
  Sum11/1 -> Sum7/2
  Sum8/1 -> Sum6/1
  Sum1/1 -> Sum5/1
  Theta Correction/1 -> Sum/1, Sum5/2, Sum6/2, Sum7/1
  Sum3/1 -> Sum/2
  Sum4/1 -> Sum11/2, Sum3/2
  Phi Correction/1 -> Sum11/1, Sum8/2, Sum1/2, Sum3/1
  Psi Correction/1 -> Sum2/2, Sum4/1
  Sum2/1 -> Sum1/1, Sum8/1

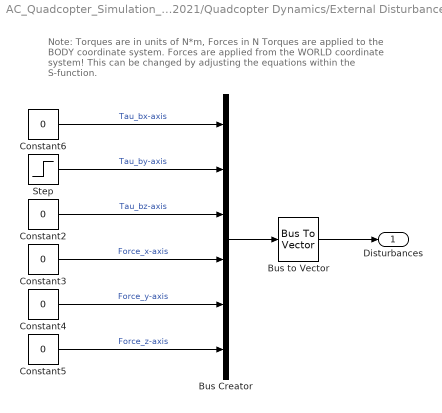
== system AC_Quadcopter_Simulation_2021/Quadcopter Dynamics/External Disturbances ==
  note: Note: Torques are in units of N*m, Forces in N
      | Torques are applied to the BODY coordinate system.
      | Forces are applied from the WORLD coordinate system!
      | This can be changed by adjusting the equations within the S-function.
  Bus Creator : BusCreator  Inputs=6
  Bus to Vector : BusToVector
  Constant{2..6} (5 alike) : Constant  Value=0
  Step : Step  After=0  SampleTime=0
  "Disturbances " : Outport
  wires:
  Constant5/1 -> Bus Creator/6  "Force_z-axis"
  Constant4/1 -> Bus Creator/5  "Force_y-axis"
  Constant3/1 -> Bus Creator/4  "Force_x-axis"
  Constant2/1 -> Bus Creator/3  "Tau_bz-axis"
  Step/1 -> Bus Creator/2  "Tau_by-axis"
  Constant6/1 -> Bus Creator/1  "Tau_bx-axis"
  Bus Creator/1 -> Bus to Vector/1
  Bus to Vector/1 -> "Disturbances "/1

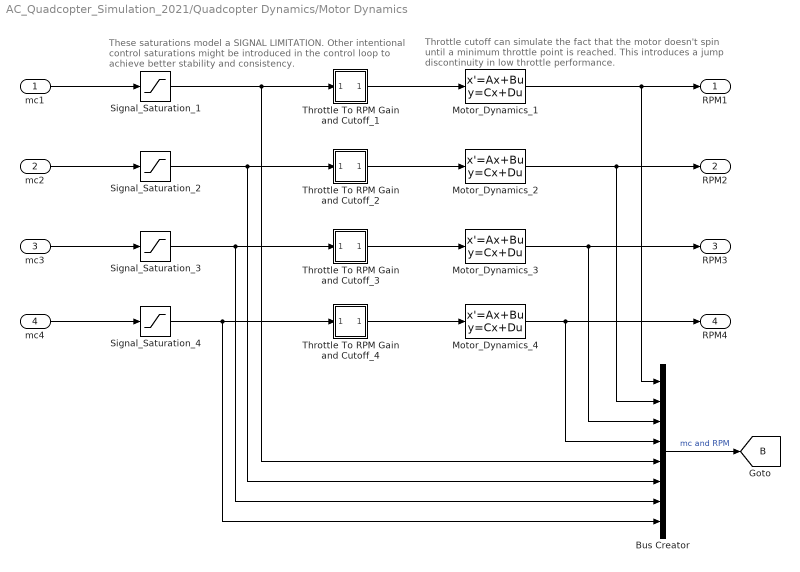
== system AC_Quadcopter_Simulation_2021/Quadcopter Dynamics/Motor Dynamics ==
  note: These saturations model a SIGNAL LIMITATION.
      | Other intentional control saturations might be introduced in the
      | control loop to achieve better stability and consistency.
  note: Throttle cutoff can simulate the fact that the motor doesn't
      | spin until a minimum throttle point is reached. This introduces
      | a jump discontinuity in low throttle performance.
  mc1 : Inport
  mc2 : Inport  Port=2
  mc3 : Inport  Port=3
  mc4 : Inport  Port=4
  Bus Creator : BusCreator  Inputs=8
  Motor_Dynamics_1 : StateSpace  A=-1/quadModel.T  C=1/quadModel.T  D=0  InitialCondition=IC.w1*quadModel.T
  Motor_Dynamics_2 : StateSpace  A=-1/quadModel.T  C=1/quadModel.T  D=0  InitialCondition=IC.w2*quadModel.T
  Motor_Dynamics_3 : StateSpace  A=-1/quadModel.T  C=1/quadModel.T  D=0  InitialCondition=IC.w3*quadModel.T
  Motor_Dynamics_4 : StateSpace  A=-1/quadModel.T  C=1/quadModel.T  D=0  InitialCondition=IC.w4*quadModel.T
  Signal_Saturation_{1..4} (4 alike) : Saturate  UpperLimit=100  LowerLimit=0
  Throttle To RPM Gain and Cutoff_1 : Subsystem
  Throttle To RPM Gain and Cutoff_2 : Subsystem
  Throttle To RPM Gain and Cutoff_3 : Subsystem
  Throttle To RPM Gain and Cutoff_4 : Subsystem
  RPM1 : Outport
  RPM2 : Outport  Port=2
  RPM3 : Outport  Port=3
  RPM4 : Outport  Port=4
  tag scope: B=global
  wires:
  Bus Creator/1 -> [B]  "mc and RPM"
  Motor_Dynamics_4/1 -> RPM4/1, Bus Creator/4
  Motor_Dynamics_3/1 -> RPM3/1, Bus Creator/3
  Motor_Dynamics_2/1 -> RPM2/1, Bus Creator/2
  Motor_Dynamics_1/1 -> RPM1/1, Bus Creator/1
  Throttle To RPM Gain and Cutoff_4/1(Out5) -> Motor_Dynamics_4/1
  Throttle To RPM Gain and Cutoff_3/1(Out5) -> Motor_Dynamics_3/1
  Throttle To RPM Gain and Cutoff_2/1(Out5) -> Motor_Dynamics_2/1
  Throttle To RPM Gain and Cutoff_1/1(Out5) -> Motor_Dynamics_1/1
  Signal_Saturation_4/1 -> Throttle To RPM Gain and Cutoff_4/1(In5), Bus Creator/8
  Signal_Saturation_3/1 -> Throttle To RPM Gain and Cutoff_3/1(In5), Bus Creator/7
  Signal_Saturation_2/1 -> Throttle To RPM Gain and Cutoff_2/1(In5), Bus Creator/6
  Signal_Saturation_1/1 -> Throttle To RPM Gain and Cutoff_1/1(In5), Bus Creator/5
  mc3/1 -> Signal_Saturation_3/1
  mc2/1 -> Signal_Saturation_2/1
  mc4/1 -> Signal_Saturation_4/1
  mc1/1 -> Signal_Saturation_1/1

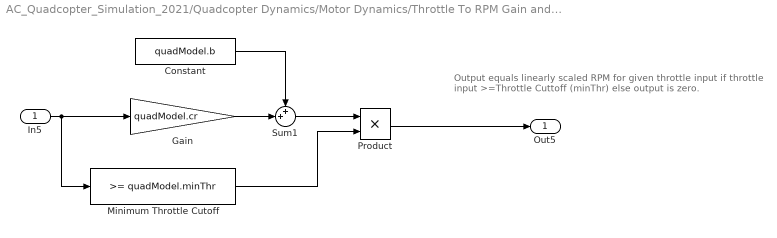
== system AC_Quadcopter_Simulation_2021/Quadcopter Dynamics/Motor Dynamics/Throttle To RPM Gain and Cutoff_1 ==
  note: Output equals linearly scaled RPM
      | for given throttle input if throttle input >=Throttle Cuttoff (minThr)
      | else output is zero.
  In5 : Inport
  Constant : Constant  Value=quadModel.b
  Gain : Gain  Gain=quadModel.cr
  Minimum Throttle Cutoff : simulink/Logic and Bit Operations/Compare To Constant  relop=>=  const=quadModel.minThr  OutDataTypeStr=uint8
  Product : Product
  Sum1 : Sum  Inputs=++|
  Out5 : Outport
  wires:
  Constant/1 -> Sum1/1
  Sum1/1 -> Product/1
  Gain/1 -> Sum1/2
  In5/1 -> Minimum Throttle Cutoff/1, Gain/1
  Product/1 -> Out5/1
  Minimum Throttle Cutoff/1 -> Product/2

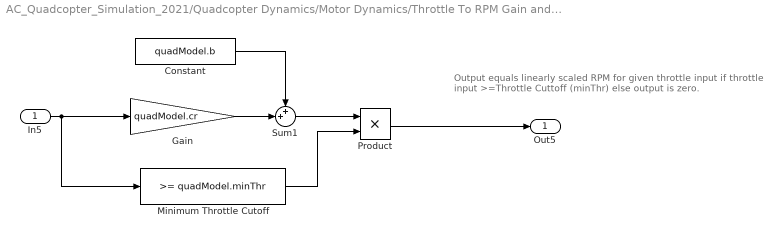
== system AC_Quadcopter_Simulation_2021/Quadcopter Dynamics/Motor Dynamics/Throttle To RPM Gain and Cutoff_2 ==
  note: Output equals linearly scaled RPM
      | for given throttle input if throttle input >=Throttle Cuttoff (minThr)
      | else output is zero.
  In5 : Inport
  Constant : Constant  Value=quadModel.b
  Gain : Gain  Gain=quadModel.cr
  Minimum Throttle Cutoff : simulink/Logic and Bit Operations/Compare To Constant  relop=>=  const=quadModel.minThr  OutDataTypeStr=uint8
  Product : Product
  Sum1 : Sum  Inputs=++|
  Out5 : Outport
  wires:
  Constant/1 -> Sum1/1
  Sum1/1 -> Product/1
  Gain/1 -> Sum1/2
  In5/1 -> Minimum Throttle Cutoff/1, Gain/1
  Product/1 -> Out5/1
  Minimum Throttle Cutoff/1 -> Product/2

== system AC_Quadcopter_Simulation_2021/Quadcopter Dynamics/Motor Dynamics/Throttle To RPM Gain and Cutoff_3 ==
  note: Output equals linearly scaled RPM
      | for given throttle input if throttle input >=Throttle Cuttoff (minThr)
      | else output is zero.
  In5 : Inport
  Constant : Constant  Value=quadModel.b
  Gain : Gain  Gain=quadModel.cr
  Minimum Throttle Cutoff : simulink/Logic and Bit Operations/Compare To Constant  relop=>=  const=quadModel.minThr  OutDataTypeStr=uint8
  Product : Product
  Sum1 : Sum  Inputs=++|
  Out5 : Outport
  wires:
  Constant/1 -> Sum1/1
  Sum1/1 -> Product/1
  Gain/1 -> Sum1/2
  In5/1 -> Minimum Throttle Cutoff/1, Gain/1
  Product/1 -> Out5/1
  Minimum Throttle Cutoff/1 -> Product/2

== system AC_Quadcopter_Simulation_2021/Quadcopter Dynamics/Motor Dynamics/Throttle To RPM Gain and Cutoff_4 ==
  note: Output equals linearly scaled RPM
      | for given throttle input if throttle input >=Throttle Cuttoff (minThr)
      | else output is zero.
  In5 : Inport
  Constant : Constant  Value=quadModel.b
  Gain : Gain  Gain=quadModel.cr
  Minimum Throttle Cutoff : simulink/Logic and Bit Operations/Compare To Constant  relop=>=  const=quadModel.minThr  OutDataTypeStr=uint8
  Product : Product
  Sum1 : Sum  Inputs=++|
  Out5 : Outport
  wires:
  Constant/1 -> Sum1/1
  Sum1/1 -> Product/1
  Gain/1 -> Sum1/2
  In5/1 -> Minimum Throttle Cutoff/1, Gain/1
  Product/1 -> Out5/1
  Minimum Throttle Cutoff/1 -> Product/2
